simulink model "penduleSimple_TP2_controle"  (R2016a)
settings: Solver=VariableStepAuto  StartTime=0.0  StopTime=200  RelTol=1e-3
values from neighbouring files (symbols this model uses):
  g = -9.81    [init.m]    (also in init_TP1.m; init_TP2_controle.m; init_tp3.m; matrices_init_tp4_partie3_4.m = 9.81)
  K = [100;10]    [init.m]    (also in init_TP2_controle.m = [20;10]; init_tp3.m = [20 10]; matrices_init_tp4_partie3_4.m = place(A,-B,V))
  l = 10    [init.m]    (also in init_TP1.m = 1; init_TP2_controle.m; init_tp3.m = 5)
  ue = 0    [init.m]    (also in init_TP2_controle.m; init_tp3.m)
  X0 = pi/4    (= 0.785398163397)    [init.m]    (also in init_TP1.m = 0.523598775598; init_TP2_controle.m; init_tp3.m = 0.628318530718)
  xe = [0;0]    [init.m]    (also in init_TP2_controle.m; init_tp3.m = [0 0])
libraries: simulink x1
settings Model: Creator=fgaribal  LastModifiedBy=fgaribal

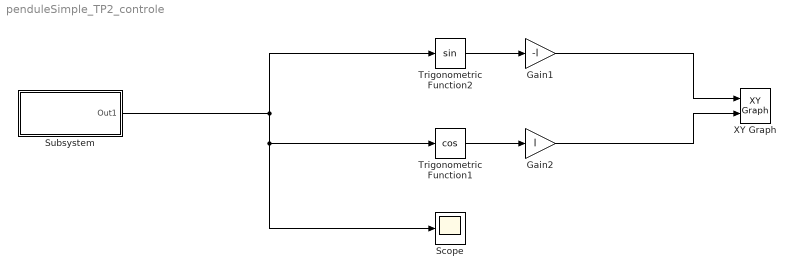
== system penduleSimple_TP2_controle ==
  Gain1 : Gain  Gain=-l
  Gain2 : Gain  Gain=l
  Scope : Scope
  Subsystem : Subsystem
  Trigonometric Function1 : Trigonometry  Operator=cos
  Trigonometric Function2 : Trigonometry
  XY Graph : simulink/Sinks/XY Graph  xmin=-l  xmax=l  ymin=-l  ymax=l  st=-1
  wires:
  Trigonometric Function1/1 -> Gain2/1
  Trigonometric Function2/1 -> Gain1/1
  Gain2/1 -> XY Graph/2
  Gain1/1 -> XY Graph/1
  Subsystem/1(Out1) -> Trigonometric Function2/1, Trigonometric Function1/1, Scope/1

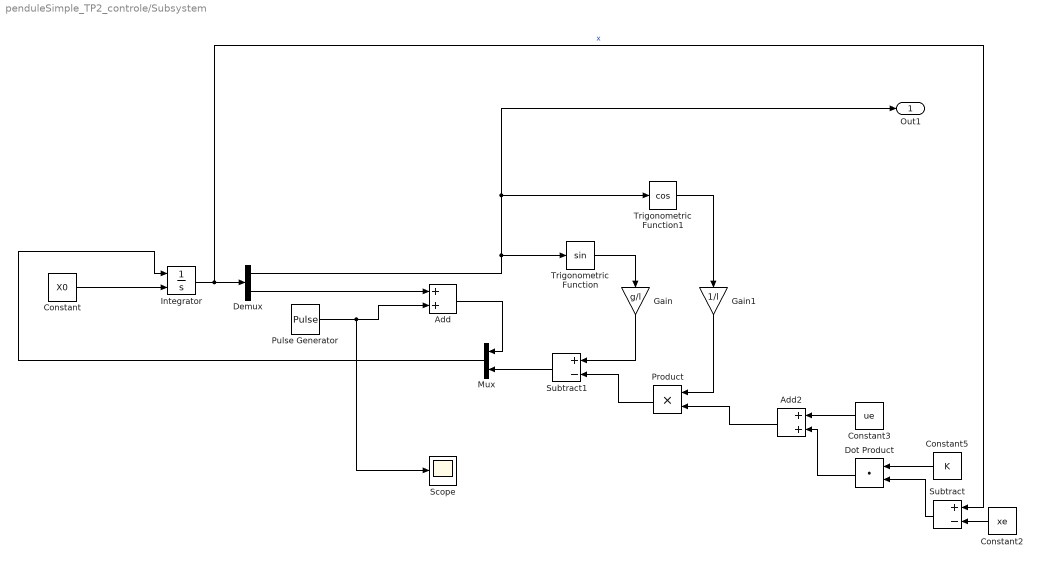
== system penduleSimple_TP2_controle/Subsystem ==
  Add : Sum
  Add2 : Sum
  Constant : Constant  Value=X0
  Constant2 : Constant  Value=xe
  Constant3 : Constant  Value=ue
  Constant5 : Constant  Value=K
  Demux : Demux  Outputs=2
  Dot Product : DotProduct  InputSameDT=on  OutDataTypeStr=Inherit: Inherit via internal rule
  Gain : Gain  Gain=g/l
  Gain1 : Gain  Gain=1/l
  Integrator : Integrator  InitialConditionSource=external
  Mux : Mux  Inputs=2
  Product : Product
  Pulse Generator : DiscretePulseGenerator  PulseType=Time based  Period=3  PulseWidth=50
  Scope : Scope
  Subtract : Sum  Inputs=+-
  Subtract1 : Sum  Inputs=+-
  Trigonometric Function : Trigonometry
  Trigonometric Function1 : Trigonometry  Operator=cos
  Out1 : Outport
  wires:
  Trigonometric Function/1 -> Gain/1
  Integrator/1 -> Subtract/1, Demux/1  "x"
  Constant/1 -> Integrator/2
  Mux/1 -> Integrator/1
  Add/1 -> Mux/1
  Pulse Generator/1 -> Scope/1, Add/2
  Demux/2 -> Add/1
  Subtract1/1 -> Mux/2
  Gain/1 -> Subtract1/1
  Constant2/1 -> Subtract/2
  Subtract/1 -> Dot Product/2
  Constant5/1 -> Dot Product/1
  Dot Product/1 -> Add2/2
  Constant3/1 -> Add2/1
  Trigonometric Function1/1 -> Gain1/1
  Demux/1 -> Out1/1, Trigonometric Function1/1, Trigonometric Function/1
  Add2/1 -> Product/2
  Gain1/1 -> Product/1
  Product/1 -> Subtract1/2
